simulink model "ssc_rankine_cycle"  (R2020b)
settings: Solver=VariableStepAuto  StartTime=0.0  StopTime=3e5  RelTol=1e-3  AbsTol=1e-3
PreLoadFcn:
  | pipe_area = 0.01; % m^2
  | furnace_temperature = 1500; % degC
  | boiler_liquid_level = 0.7; % 1
  | condenser_liquid_level = 0.2;
  | preheat_condenser_liquid_level = 0.2; % 1
undefined symbols (not defined in the file): sigbuilder_block
libraries: fl_lib x50, nesl_utility x18, RankineCycle_lib x5, pid_lib x2
(part 1 of 3)
CloseFcn:
  | try,close(h1_ssc_rankine_cycle),end
  | clear h1_ssc_rankine_cycle
  | try,close(h2_ssc_rankine_cycle),end
  | clear h2_ssc_rankine_cycle
  | try,close(h3_ssc_rankine_cycle),end
  | clear h3_ssc_rankine_cycle
  | 
  | clear simlog_ssc_rankine_cycle tout
  | clear pipe_area furnace_temperature boiler_liquid_level condenser_liquid_level preheat_condenser_liquid_level
Description:
  | Rankine Cycle (Steam Turbine)
settings Model: Creator=The MathWorks, Inc.  LastModifiedBy=Destiny-Zhu
settings SolverCC: AutoScaleAbsTol=off  MaxConsecutiveMinStep=2
settings DataIOCC: LimitDataPoints=on  MaxDataPoints=10000  ReturnWorkspaceOutputs=off
settings DebuggingCC: PregeneratedLibrarySubsystemCodeDiagnostic=none  ArithmeticOperatorsInVariantConditions=warning
settings SFSimCC: SimUseLocalCustomCode=off  CustomCodeUndefinedFunction=UseInterfaceOnly
settings RTWCC: RTWUseLocalCustomCode=off
settings CodeAppCC: StateflowObjectComments=on
settings SimscapeCC: SimscapeLogType=all  SimscapeLogSimulationStatistics=on  SimscapeLogName=simlog_ssc_rankine_cycle  SimscapeLogDataHistory=10000

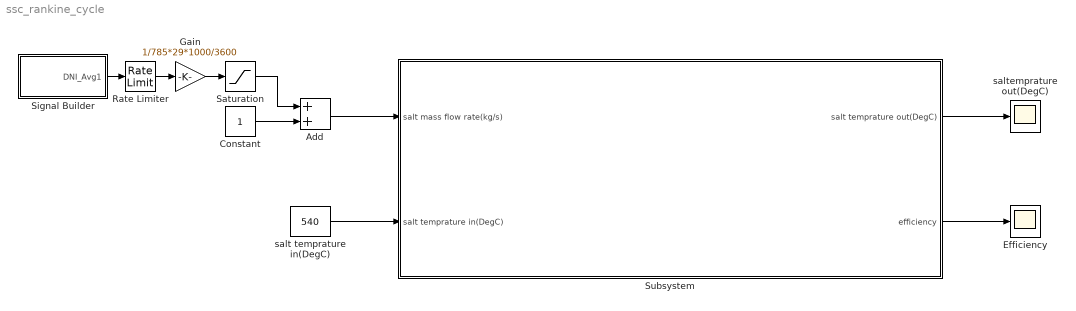
== system ssc_rankine_cycle ==
  Add : Sum
  Constant : Constant
  Efficiency : Scope
  Gain : Gain  Gain=1/785*29*1000/3600
  Rate Limiter : RateLimiter  RisingSlewLimit=10  FallingSlewLimit=-10  SampleTimeMode=inherited
  Saturation : Saturate  UpperLimit=1000  LowerLimit=0
  Signal Builder : Subsystem  Tag=STV Subsys  LoadFcn=sigbuilder_block('load');  StartFcn=sigbuilder_block('start');  StopFcn=sigbuilder_block('stop');  ClipboardFcn=sigbuilder_block('clipboard');  mask(Sigbuilder block){tuvar=[0:10]}
      mask help: Simulink:masks:SigbuilderBlock_MD
      mask init:
      | if ~strcmp(get_param(bdroot(gcbh),'SimulationStatus'),'stopped') tuvar = sigbuilder_block('maskInit'); end
      settings: CopyFcn=sigbuilder_block('copy');  DeleteFcn=sigbuilder_block('delete');  ModelCloseFcn=sigbuilder_block('modelClose');  PreSaveFcn=sigbuilder_block('preSave');  PauseFcn=sigbuilder_block('pause');  ContinueFcn=sigbuilder_block('continue');  NameChangeFcn=sigbuilder_block('namechange');  OpenFcn=sigbuilder_block('open',[151.5 202.875 550.5 400.125 ]);  CloseFcn=sigbuilder_block('close');
      mask Display: plot(0, 0, 100, 100,[2, 2, 32, 32, 2], [68, 8, 8, 68, 68],[32, 2], [38, 38], [32, 19, 2],[53, 60, 44], [32, 17, 17, 2],[16, 16, 31, 31]);txt = getActiveGroup(gcbh);text(2, 100, txt,'verticalAlignment', 'top');
  Subsystem : Subsystem
  salt temprature in(DegC) : Constant  Value=540
  saltemprature out(DegC) : Scope
  wires:
  Add/1 -> Subsystem/1(salt mass flow rate(kg/s))
  salt temprature in(DegC)/1 -> Subsystem/2(salt temprature in(DegC))
  Subsystem/1(salt temprature out(DegC)) -> saltemprature out(DegC)/1
  Signal Builder/1(DNI_Avg1) -> Rate Limiter/1
  Rate Limiter/1 -> Gain/1
  Gain/1 -> Saturation/1
  Constant/1 -> Add/2
  Saturation/1 -> Add/1
  Subsystem/2(efficiency) -> Efficiency/1

== system ssc_rankine_cycle/Signal Builder ==
  Demux : Demux  Tag=STV Demux  Outputs=1
      settings: DisplayOption=none
  FromWs : FromWorkspace  Tag=STV FromWs  VariableName=tuvar
      SigBuilderData=|
      | common.afterFinalStr = 'Extrapolate'
      | common.sampleTime = 0
      | dataSet.timeRange = [0 259260]
      | dataSet.name = 'Group 1'
      | sbobj.Groups.Name = 'Group 1'
      | sbobj.Groups.Signals.Name = 'DNI_Avg1'
      | sbobj.Groups.Signals.XData = [0 60 120 180 240 300 360 420 480 540 600 660 ... (4322 elements, 1x4322)]
      | sbobj.Groups.Signals.YData = [-2.093828 0.820727 -1.83532 -1.790075 -2.694803 -2.151961 1.518648 -0.6850063 1.628504 0.8336399 -0.05816128 0.05816069 ... (4322 elements, 1x4322)]
      | sbobj.Groups.TimeRange = [0 259260]
  DNI_Avg1 : Outport  Tag=STV Outport
  wires:
  FromWs/1 -> Demux/1
  Demux/1 -> DNI_Avg1/1
